simulink model "shuntconverterlms1"  (R2018a)
settings: Solver=VariableStepAuto  StartTime=0.0  StopTime=1  RelTol=1e-3
libraries: powerlib x20, eeGeneralControl x4, simulink x2
settings Model: Creator=sanje  LastModifiedBy=sanje
settings DataIOCC: ReturnWorkspaceOutputs=on
settings SFSimCC: SimUseLocalCustomCode=on
settings RTWCC: RTWUseLocalCustomCode=on

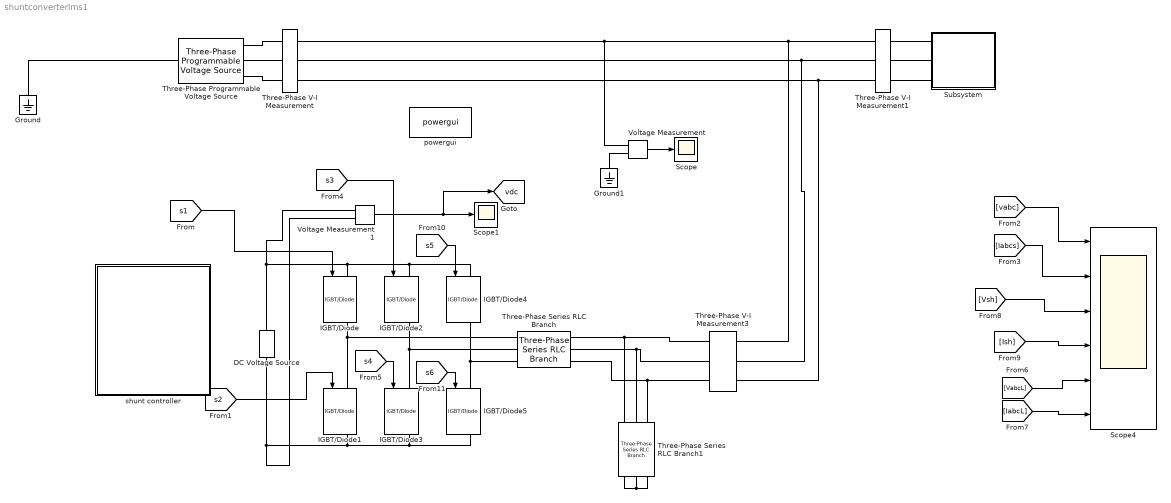
== system shuntconverterlms1 ==
  DC Voltage Source : powerlib/Electrical Sources/DC Voltage Source  Amplitude=700  Measurements=None
      settings: SourceProductName=Simscape Electrical
  Ground : powerlib/Elements/Ground  LConnTagsString=a
      settings: SourceProductName=Simscape Electrical
  Ground1 : powerlib/Elements/Ground  LConnTagsString=a
      settings: SourceProductName=Simscape Electrical
  IGBT/Diode{,1..5} (6 alike) : powerlib/Power Electronics/IGBT//Diode  Ron=1e-3  Rs=1e5  Cs=inf  Measurements=on
      settings: SourceProductName=Simscape Electrical
  Scope : Scope
  Scope1 : Scope
  Scope4 : Scope  NumInputPorts=6
  Subsystem : Subsystem
  Three-Phase Programmable Voltage Source : powerlib/Electrical Sources/Three-Phase Programmable Voltage Source  PositiveSequence="[415  0 50]"  VariationEntity=None  VariationType=Table of time-amplitude pairs  VariationTypeAlt=Step  VariationStep=0.5  VariationRate=10  VariationMagnitude=0.3  VariationFrequency=2  VariationTiming=[1 2]  VariationPhaseA=off  Amplitudes=[1 0.8 1 1.2 1.0]  TimeValues=[0 0.1 0.15 0.2 0.25]  HarmonicGeneration=off  HarmonicA=[3 0.2 -25 0]  HarmonicB=[2 0.15 35 2]  Timing="[0.05  3]"  BusType=swing  Pref=0  Qref=0  Qmin=-inf  Qmax=inf
      settings: SourceProductName=Simscape Electrical
  Three-Phase Series RLC Branch : powerlib/Elements/Three-Phase Series RLC Branch  LConnTagsString=A|B|C  RConnTagsString=A|B|C  BranchType=L  Resistance=1  Inductance=2.5e-3  Capacitance=1e-6  Measurements=None
      settings: SourceProductName=Simscape Electrical
  Three-Phase Series RLC Branch1 : powerlib/Elements/Three-Phase Series RLC Branch  LConnTagsString=A|B|C  RConnTagsString=A|B|C  BranchType=RC  Resistance=5  Inductance=1e-3  Capacitance=10e-6  Measurements=None
      settings: SourceProductName=Simscape Electrical
  Three-Phase V-I Measurement : powerlib/Measurements/Three-Phase V-I Measurement  VoltageMeasurement=phase-to-ground  SetLabelV=on  LabelV=vabc  Vpu=off  VpuLL=off  CurrentMeasurement=yes  SetLabelI=on  LabelI=Iabcs  Ipu=off  Pbase=100e6  Vbase=500e3  OutputType=Complex  PhasorSimulation=off  PSBequivalent=0
      settings: SourceProductName=Simscape Electrical
  Three-Phase V-I Measurement1 : powerlib/Measurements/Three-Phase V-I Measurement  VoltageMeasurement=phase-to-ground  SetLabelV=on  LabelV=VabcL  Vpu=off  VpuLL=off  CurrentMeasurement=yes  SetLabelI=on  LabelI=IabcL  Ipu=off  Pbase=100e6  Vbase=500e3  OutputType=Complex  PhasorSimulation=off  PSBequivalent=0
      settings: SourceProductName=Simscape Electrical
  Three-Phase V-I Measurement3 : powerlib/Measurements/Three-Phase V-I Measurement  VoltageMeasurement=phase-to-ground  SetLabelV=on  LabelV=Vsh  Vpu=off  VpuLL=off  CurrentMeasurement=yes  SetLabelI=on  LabelI=Ish  Ipu=off  Pbase=100e6  Vbase=500e3  OutputType=Complex  PhasorSimulation=off  PSBequivalent=0
      settings: SourceProductName=Simscape Electrical
  Voltage Measurement : powerlib/Measurements/Voltage Measurement  PhasorSimulation=off  OutputType=Complex  PSBequivalent=0
      settings: SourceProductName=Simscape Electrical
  Voltage Measurement1 : powerlib/Measurements/Voltage Measurement  PhasorSimulation=off  OutputType=Complex  PSBequivalent=0
      settings: SourceProductName=Simscape Electrical
  powergui : powerlib/powergui  Priority=1  SimulationMode=Discrete  SampleTime=10e-6  frequency=60  Iterations=50  frequencyindice=0  Pbase=100e6  ErrMax=1e-4  UnitsV=kV  UnitsW=MW  buscounter=0  FunctionMessages=off  echomessages=off  EnableUseOfTLC=off  CurrentSourceSwitches=off  DisableSnubberDevices=off  DisableRonSwitches=off  DisableVfSwitches=off  DisplayEquations=off  AutomaticDiscreteSolvers=off  SolverType=Tustin/Backward Euler (TBE)  Interpol=off  ExternalGateDelay=off  methode=off  Ts=100  x0status=blocks  SPID=on  SwTol=0  HookPort=off  NonlinearTolerance=1e-4  nMaxIteration=100  ContinueOnMaxIteration=off  RestoreLinks=warning  ResistiveCurrentMeasurement=off  Frange=[0:2:500]  Ylog=off  Xlog=on  ShowGrid=off  save=off  variable=ZData  structure=0  ZoomFFT=off  StartTime=0.0  cycles=1  DisplayStyle=1  fundamental=60  FreqAxis=off  MaxFrequency=1000  frequencyindicesteady=1  RmsSteady=1  display=off
      settings: SourceProductName=Simscape Electrical
  shunt controller : Subsystem
  tag scope: vdc=global
  wires:
  [Iabcs] -> Scope4/2
  [vabc] -> Scope4/1
  Voltage Measurement/1 -> Scope/1
  Voltage Measurement1/1 -> Scope1/1, [vdc]
  [Vsh] -> Scope4/3
  [VabcL] -> Scope4/5
  [IabcL] -> Scope4/6
  [Ish] -> Scope4/4
  [s1] -> IGBT/Diode/1
  [s2] -> IGBT/Diode1/1
  [s3] -> IGBT/Diode2/1
  [s4] -> IGBT/Diode3/1
  [s5] -> IGBT/Diode4/1
  [s6] -> IGBT/Diode5/1
  connections:
  Three-Phase Programmable Voltage Source/RConn1 -- Three-Phase V-I Measurement/LConn1
  Subsystem/LConn1 -- Three-Phase V-I Measurement1/RConn1
  Subsystem/LConn3 -- Three-Phase V-I Measurement1/RConn3
  Subsystem/LConn2 -- Three-Phase V-I Measurement1/RConn2
  Three-Phase Programmable Voltage Source/RConn3 -- Three-Phase V-I Measurement/LConn3
  Ground/LConn1 -- Three-Phase Programmable Voltage Source/LConn1
  Three-Phase V-I Measurement/LConn2 -- Three-Phase Programmable Voltage Source/RConn2
  Three-Phase V-I Measurement1/LConn1 -- Three-Phase V-I Measurement3/RConn1 -- Voltage Measurement/LConn1 -- Three-Phase V-I Measurement/RConn1
  Three-Phase V-I Measurement1/LConn2 -- Three-Phase V-I Measurement3/RConn2 -- Three-Phase V-I Measurement/RConn2
  Three-Phase V-I Measurement1/LConn3 -- Three-Phase V-I Measurement3/RConn3 -- Three-Phase V-I Measurement/RConn3
  Three-Phase Series RLC Branch/LConn2 -- Three-Phase Series RLC Branch1/RConn2 -- Three-Phase V-I Measurement3/LConn2
  Three-Phase Series RLC Branch/LConn3 -- Three-Phase Series RLC Branch1/RConn3 -- Three-Phase V-I Measurement3/LConn3
  Three-Phase Series RLC Branch/LConn1 -- Three-Phase Series RLC Branch1/RConn1 -- Three-Phase V-I Measurement3/LConn1
  Ground1/LConn1 -- Voltage Measurement/LConn2
  Three-Phase Series RLC Branch1/LConn1 -- Three-Phase Series RLC Branch1/LConn3 -- Three-Phase Series RLC Branch1/LConn2
  IGBT/Diode1/LConn1 -- Three-Phase Series RLC Branch/RConn1 -- IGBT/Diode/RConn1
  IGBT/Diode4/RConn1 -- IGBT/Diode5/LConn1 -- Three-Phase Series RLC Branch/RConn3
  IGBT/Diode2/RConn1 -- IGBT/Diode3/LConn1 -- Three-Phase Series RLC Branch/RConn2
  DC Voltage Source/RConn1 -- IGBT/Diode4/LConn1 -- IGBT/Diode2/LConn1 -- IGBT/Diode/LConn1 -- Voltage Measurement1/LConn1
  DC Voltage Source/LConn1 -- Voltage Measurement1/LConn2 -- IGBT/Diode5/RConn1 -- IGBT/Diode3/RConn1 -- IGBT/Diode1/RConn1

== system shuntconverterlms1/Subsystem ==
  Series RLC Branch11 : powerlib/Elements/Series RLC Branch  LConnTagsString=__new0  RConnTagsString=__new0  BranchType=RL  Resistance=11  Inductance=120e-3  SetiL0=off  InitialCurrent=0  Capacitance=1e-6  Setx0=off  InitialVoltage=0  Measurements=None
      settings: SourceProductName=Simscape Electrical
  Universal Bridge : powerlib/Power Electronics/Universal Bridge  Arms=3  SnubberResistance=1e5  SnubberCapacitance=inf  Device=Diodes  Ron=1e-3  Lon=0  ForwardVoltages="[  0  0  ]"  ForwardVoltage=0  GTOparameters=[ 10e-6 , 20e-6 ]  IGBTparameters=[ 1e-6 , 2e-6 ]  Measurements=None  Measurements_2=None  converterType=Rectifier
      settings: SourceProductName=Simscape Electrical
  Conn1 : PMIOPort  Side=Left
  Conn4 : PMIOPort  Port=2  Side=Left
  Conn2 : PMIOPort  Port=3  Side=Left
  connections:
  Universal Bridge/RConn2 -- Series RLC Branch11/RConn1
  Universal Bridge/RConn1 -- Series RLC Branch11/LConn1
  Conn1/RConn1 -- Universal Bridge/LConn1
  Conn2/RConn1 -- Universal Bridge/LConn3
  Universal Bridge/LConn2 -- Conn4/RConn1

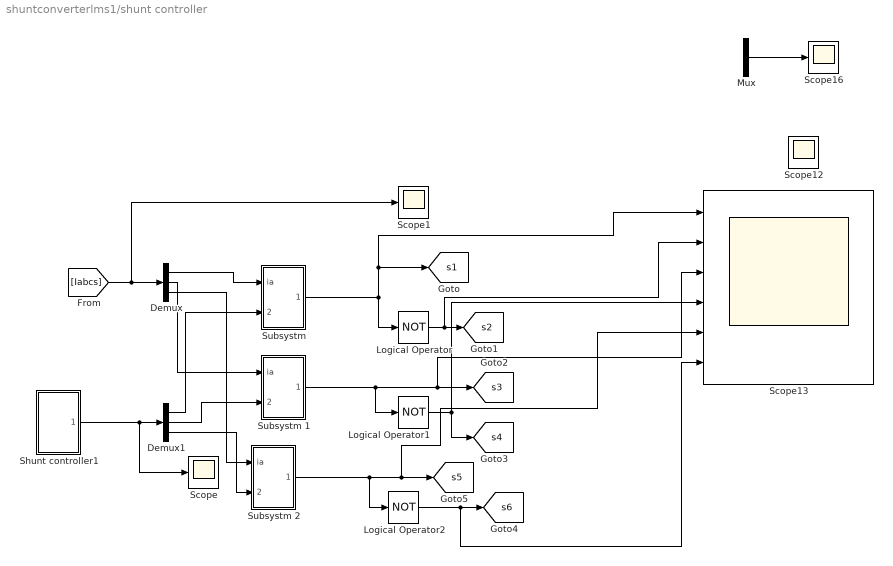
== system shuntconverterlms1/shunt controller ==
  Demux : Demux  Outputs=3
  Demux1 : Demux  Outputs=3
  Logical Operator : Logic  Operator=NOT  AllPortsSameDT=off  OutDataTypeStr=boolean
  Logical Operator1 : Logic  Operator=NOT  AllPortsSameDT=off  OutDataTypeStr=boolean
  Logical Operator2 : Logic  Operator=NOT  AllPortsSameDT=off  OutDataTypeStr=boolean
  Mux : Mux  Inputs=3
  Scope{,1,12,16} (4 alike) : Scope
  Scope13 : Scope  NumInputPorts=6
  Shunt controller1 : Subsystem
  "Subsystm " : Subsystem
  Subsystm 1 : Subsystem
  Subsystm 2 : Subsystem
  tag scope: s1=global, s2=global, s3=global, s4=global, s5=global, s6=global
  wires:
  Mux/1 -> Scope16/1
  Shunt controller1/1(Outport) -> Scope/1, Demux1/1
  [Iabcs] -> Scope1/1, Demux/1
  Demux/1 -> "Subsystm "/1(ia)
  Demux1/1 -> "Subsystm "/2(In2)
  Demux/2 -> Subsystm 1/1(ia)
  Demux1/2 -> Subsystm 1/2(In2)
  Demux/3 -> Subsystm 2/1(ia)
  Demux1/3 -> Subsystm 2/2(In2)
  "Subsystm "/1(Out1) -> Logical Operator/1, Scope13/1, [s1]
  Subsystm 1/1(Out1) -> Scope13/3, [s3], Logical Operator1/1
  Subsystm 2/1(Out1) -> Scope13/5, [s5], Logical Operator2/1
  Logical Operator/1 -> Scope13/2, [s2]
  Logical Operator1/1 -> [s4], Scope13/4
  Logical Operator2/1 -> Scope13/6, [s6]

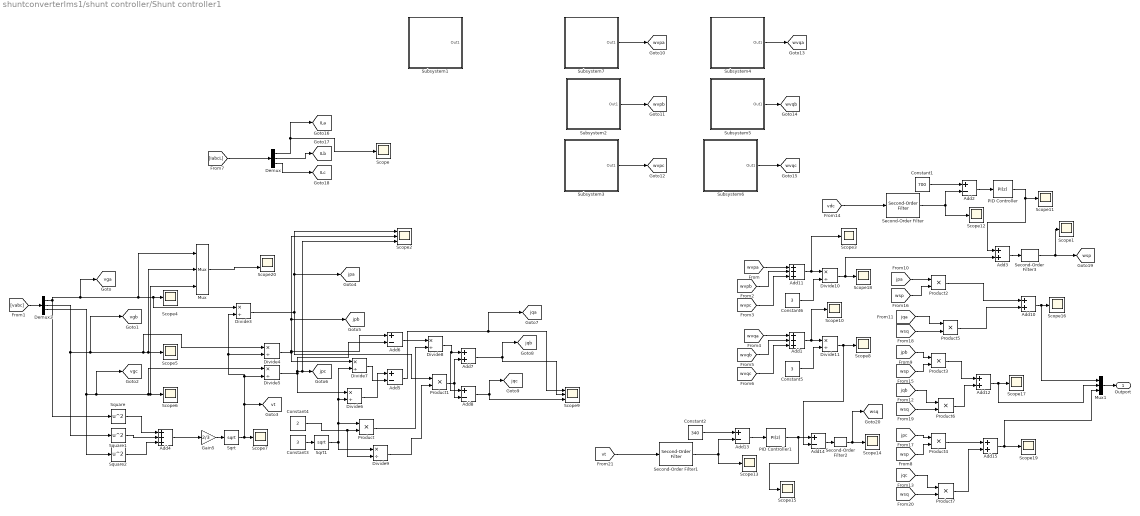
== system shuntconverterlms1/shunt controller/Shunt controller1 ==
  Add1 : Sum  Inputs=+++
  Add{3,7,10,12,15} (5 alike) : Sum
  Add11 : Sum  Inputs=+++
  Add{2,5..6,8,13..14} (6 alike) : Sum  Inputs=+-
  Add4 : Sum  Inputs=+++
  Constant1 : Constant  Value=700
  Constant2 : Constant  Value=340
  Constant3 : Constant  Value=3
  Constant4 : Constant  Value=2
  Constant5 : Constant  Value=3
  Constant6 : Constant  Value=3
  Demux : Demux  Outputs=3
  Demux2 : Demux  Outputs=3
  Divide{3..11} (9 alike) : Product  Inputs=*/
  Gain5 : Gain  Gain=2/3
  Mux : Mux  Inputs=3
  Mux1 : Mux  Inputs=3
  PID Controller : simulink/Continuous/PID Controller  Controller=PI  Form=Parallel  TimeDomain=Discrete-time  SampleTime=-1  IntegratorMethod=Forward Euler  FilterMethod=Forward Euler  ControllerParametersSource=internal  P=1  I=1  D=0  UseFilter=on  N=100  TunerSelectOption=Transfer Function Based (PID Tuner App)  InitialConditionSource=internal  InitialConditionForIntegrator=0  InitialConditionForFilter=0  DifferentiatorICPrevScaledInput=0  ExternalReset=none  TrackingMode=off  Kt=1  LimitOutput=off  UpperSaturationLimit=inf  LowerSaturationLimit=-inf  LinearizeAsGain=on  AntiWindupMode=none  Kb=1  POutMin=[]  POutMax=[]  IOutMin=[]  IOutMax=[]  DOutMin=[]  DOutMax=[]  NOutMin=[]  NOutMax=[]  SumOutMin=[]  SumOutMax=[]  SaturationOutMin=[]  SaturationOutMax=[]  PParamMin=[]  PParamMax=[]  IParamMin=[]  IParamMax=[]  DParamMin=[]  DParamMax=[]  NParamMin=[]  NParamMax=[]  KbParamMin=[]  KbParamMax=[]  KtParamMin=[]  KtParamMax=[]  KbOutMin=[]  KbOutMax=[]  KtOutMin=[]  KtOutMax=[]  IntegratorOutMin=[]  IntegratorOutMax=[]  FilterOutMin=[]  FilterOutMax=[]  SumI1OutMin=[]  SumI1OutMax=[]  SumI2OutMin=[]  SumI2OutMax=[]  SumI3OutMin=[]  SumI3OutMax=[]  SumDOutMin=[]  SumDOutMax=[]  DifferentiatorOutMin=[]  DifferentiatorOutMax=[]  FilterDiffOutCoefMin=[]  FilterDiffOutCoefMax=[]  ReciprocalOutMin=[]  ReciprocalOutMax=[]  SumDenOutMin=[]  SumDenOutMax=[]  SumNumOutMin=[]  SumNumOutMax=[]  DivideOutMin=[]  DivideOutMax=[]  IntegratorContinuousStateAttributes=''  IntegratorStateMustResolveToSignalObject=off  IntegratorRTWStateStorageClass=Auto  FilterContinuousStateAttributes=''  FilterStateMustResolveToSignalObject=off  FilterRTWStateStorageClass=Auto
  PID Controller1 : simulink/Continuous/PID Controller  Controller=PI  Form=Parallel  TimeDomain=Discrete-time  SampleTime=-1  IntegratorMethod=Forward Euler  FilterMethod=Forward Euler  ControllerParametersSource=internal  P=1  I=1  D=0  UseFilter=on  N=100  TunerSelectOption=Transfer Function Based (PID Tuner App)  InitialConditionSource=internal  InitialConditionForIntegrator=0  InitialConditionForFilter=0  DifferentiatorICPrevScaledInput=0  ExternalReset=none  TrackingMode=off  Kt=1  LimitOutput=off  UpperSaturationLimit=inf  LowerSaturationLimit=-inf  LinearizeAsGain=on  AntiWindupMode=none  Kb=1  POutMin=[]  POutMax=[]  IOutMin=[]  IOutMax=[]  DOutMin=[]  DOutMax=[]  NOutMin=[]  NOutMax=[]  SumOutMin=[]  SumOutMax=[]  SaturationOutMin=[]  SaturationOutMax=[]  PParamMin=[]  PParamMax=[]  IParamMin=[]  IParamMax=[]  DParamMin=[]  DParamMax=[]  NParamMin=[]  NParamMax=[]  KbParamMin=[]  KbParamMax=[]  KtParamMin=[]  KtParamMax=[]  KbOutMin=[]  KbOutMax=[]  KtOutMin=[]  KtOutMax=[]  IntegratorOutMin=[]  IntegratorOutMax=[]  FilterOutMin=[]  FilterOutMax=[]  SumI1OutMin=[]  SumI1OutMax=[]  SumI2OutMin=[]  SumI2OutMax=[]  SumI3OutMin=[]  SumI3OutMax=[]  SumDOutMin=[]  SumDOutMax=[]  DifferentiatorOutMin=[]  DifferentiatorOutMax=[]  FilterDiffOutCoefMin=[]  FilterDiffOutCoefMax=[]  ReciprocalOutMin=[]  ReciprocalOutMax=[]  SumDenOutMin=[]  SumDenOutMax=[]  SumNumOutMin=[]  SumNumOutMax=[]  DivideOutMin=[]  DivideOutMax=[]  IntegratorContinuousStateAttributes=''  IntegratorStateMustResolveToSignalObject=off  IntegratorRTWStateStorageClass=Auto  FilterContinuousStateAttributes=''  FilterStateMustResolveToSignalObject=off  FilterRTWStateStorageClass=Auto
  Product{,1..7} (8 alike) : Product
  Scope{,1,3..8,10..19} (18 alike) : Scope
  Scope2 : Scope  NumInputPorts=3
  Scope20 : Scope  NumInputPorts=2
  Scope9 : Scope  NumInputPorts=3
  Second-Order Filter : eeGeneralControl/Second-Order Filter  FilterType=Low-pass  fn=50  Zeta=0.707  Ts=10e-6  A0=0  Ph0=0  f0=0  b0=0
      settings: SourceProductName=Simscape Electrical  SourceProductBaseCode=PS
  Second-Order Filter1 : eeGeneralControl/Second-Order Filter  FilterType=Low-pass  fn=50  Zeta=0.707  Ts=10e-6  A0=0  Ph0=0  f0=0  b0=0
      settings: SourceProductName=Simscape Electrical  SourceProductBaseCode=PS
  Second-Order Filter2 : eeGeneralControl/Second-Order Filter  FilterType=Low-pass  fn=10  Zeta=0.707  Ts=10e-6  A0=0  Ph0=0  f0=0  b0=0
      settings: SourceProductName=Simscape Electrical  SourceProductBaseCode=PS
  Second-Order Filter3 : eeGeneralControl/Second-Order Filter  FilterType=Low-pass  fn=10  Zeta=0.707  Ts=10e-6  A0=0  Ph0=0  f0=0  b0=0
      settings: SourceProductName=Simscape Electrical  SourceProductBaseCode=PS
  Sqrt : Sqrt  SaturateOnIntegerOverflow=on
  Sqrt1 : Sqrt  SaturateOnIntegerOverflow=on
  Square : Math  Operator=square  SaturateOnIntegerOverflow=on
  Square1 : Math  Operator=square  SaturateOnIntegerOverflow=on
  Square2 : Math  Operator=square  SaturateOnIntegerOverflow=on
  Subsystem1 : Subsystem
  Subsystem2 : Subsystem
  Subsystem3 : Subsystem
  Subsystem4 : Subsystem
  Subsystem5 : Subsystem
  Subsystem6 : Subsystem
  Subsystem7 : Subsystem
  Outport : Outport
  tag scope: ILa=global, ILb=global, ILc=global, jpa=global, jpb=global, jpc=global, jqa=global, jqb=global, jqc=global, vga=global, vgb=global, vgc=global, vt=global, wsp=global, wsq=global, wvpa=global, wvpb=global, wvpc=global, wvqa=global, wvqb=global, wvqc=global
  wires:
  Add6/1 -> Divide8/1
  Constant4/1 -> Divide9/2, Product/2
  Constant3/1 -> Sqrt1/1
  Add8/1 -> [jqc], Scope9/3
  Product/1 -> Divide8/2
  Divide5/1 -> Add6/2, Scope2/3, [jpc], Divide6/1
  Divide4/1 -> Divide7/1, Scope2/2, [jpb], Add6/1
  Square1/1 -> Add4/2
  Add7/1 -> [jqb], Scope9/2
  Divide8/1 -> Add7/1, Add8/1
  Product1/1 -> Add8/2, Add7/2
  Mux/1 -> Scope20/2
  Divide7/1 -> Add5/2
  Divide9/1 -> Product1/2
  Sqrt1/1 -> Product/1, Divide7/2, Divide6/2, Divide9/1
  Divide6/1 -> Add5/1
  Square/1 -> Add4/1
  Add4/1 -> Gain5/1
  Sqrt/1 -> Divide5/2, Divide4/2, Divide3/2, [vt], Scope7/1
  Gain5/1 -> Sqrt/1
  Divide3/1 -> Product1/1, Scope2/1, [jpa]
  Demux2/2 -> Square1/1, [vgb], Mux/2, Scope5/1, Divide4/1
  Demux2/1 -> [vga], Mux/1, Divide3/1, Scope4/1, Square/1
  Square2/1 -> Add4/3
  Demux2/3 -> Square2/1, [vgc], Mux/3, Scope6/1, Divide5/1
  Add5/1 -> [jqa], Scope9/1
  [vabc] -> Demux2/1
  [wvpb] -> Add11/2
  [wvqa] -> Add1/1
  [wvqb] -> Add1/2
  Subsystem4/1(Out1) -> [wvqa]
  Subsystem3/1(Out1) -> [wvpc]
  [wvqc] -> Add1/3
  [wvpc] -> Add11/3
  Add11/1 -> Scope3/1, Divide10/1
  Add1/1 -> Scope10/1, Divide11/1
  Subsystem5/1(Out1) -> [wvqb]
  Divide10/1 -> Add3/2, Scope18/1
  Subsystem2/1(Out1) -> [wvpb]
  [wvpa] -> Add11/1
  Constant6/1 -> Divide10/2
  Subsystem7/1(Out1) -> [wvpa]
  Constant5/1 -> Divide11/2
  Subsystem6/1(Out1) -> [wvqc]
  Divide11/1 -> Add14/2, Scope8/1
  [IabcL] -> Demux/1
  Demux/1 -> [ILa], Scope/1
  Demux/2 -> [ILb]
  Demux/3 -> [ILc]
  Constant1/1 -> Add2/1
  [vdc] -> Second-Order Filter/1
  Second-Order Filter/1 -> Add2/2, Scope12/1
  Add2/1 -> PID Controller/1
  PID Controller/1 -> Add3/1, Scope11/1
  [jpa] -> Product2/1
  [wsp] -> Product2/2
  [jpb] -> Product3/1
  [wsp] -> Product3/2
  [jpc] -> Product4/1
  [wsp] -> Product4/2
  [wsq] -> Product5/2
  [jqa] -> Product5/1
  [jqb] -> Product6/1
  [wsq] -> Product6/2
  [wsq] -> Product7/2
  [jqc] -> Product7/1
  Product2/1 -> Add10/1
  Product5/1 -> Add10/2
  Product3/1 -> Add12/1
  Product6/1 -> Add12/2
  PID Controller1/1 -> Scope15/1, Add14/1
  Add13/1 -> PID Controller1/1
  Second-Order Filter1/1 -> Scope13/1, Add13/2
  [vt] -> Second-Order Filter1/1
  Constant2/1 -> Add13/1
  Add14/1 -> Second-Order Filter2/1
  Product4/1 -> Add15/1
  Product7/1 -> Add15/2
  Add10/1 -> Mux1/1, Scope16/1
  Add12/1 -> Mux1/2, Scope17/1
  Add15/1 -> Mux1/3, Scope19/1
  Mux1/1 -> Outport/1
  Second-Order Filter2/1 -> [wsq], Scope14/1
  Add3/1 -> Second-Order Filter3/1
  Second-Order Filter3/1 -> Scope1/1, [wsp]

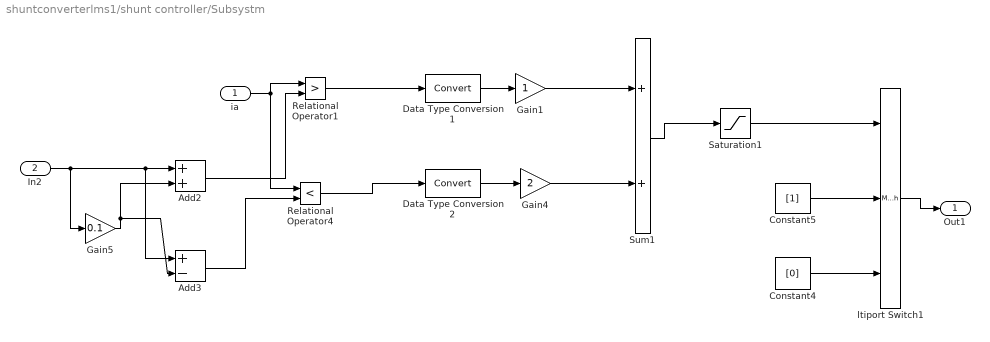
== system shuntconverterlms1/shunt controller/Subsystm  ==
  ia : Inport
  In2 : Inport  Port=2
  Add2 : Sum
  Add3 : Sum  Inputs=+-
  Constant4 : Constant  Value=[0]
  Constant5 : Constant  Value=[1]
  Data Type Conversion1 : DataTypeConversion  SaturateOnIntegerOverflow=on  RndMeth=Zero
  Data Type Conversion2 : DataTypeConversion  SaturateOnIntegerOverflow=on  RndMeth=Zero
  Gain1 : Gain  SaturateOnIntegerOverflow=on  OutDataTypeStr=Inherit: Same as input  ParamDataTypeStr=Inherit: Same as input
  Gain4 : Gain  Gain=2  SaturateOnIntegerOverflow=on  OutDataTypeStr=Inherit: Same as input  ParamDataTypeStr=Inherit: Same as input
  Gain5 : Gain  Gain=0.1
  Relational Operator1 : RelationalOperator  Operator=>  RndMeth=Nearest  InputSameDT=on
  Relational Operator4 : RelationalOperator  Operator=<  RndMeth=Nearest  InputSameDT=on
  Saturation1 : Saturate  UpperLimit=2  LowerLimit=1
  Sum1 : Sum  SaturateOnIntegerOverflow=on  InputSameDT=on  OutDataTypeStr=Inherit: Same as first input
  ltiport Switch1 : MultiPortSwitch  Inputs=2
  Out1 : Outport
  wires:
  In2/1 -> Add3/1, Add2/1, Gain5/1
  Data Type Conversion2/1 -> Gain4/1
  Data Type Conversion1/1 -> Gain1/1
  Relational Operator1/1 -> Data Type Conversion1/1
  Relational Operator4/1 -> Data Type Conversion2/1
  ia/1 -> Relational Operator4/1, Relational Operator1/1
  Gain5/1 -> Add2/2, Add3/2
  Add2/1 -> Relational Operator1/2
  Add3/1 -> Relational Operator4/2
  Saturation1/1 -> ltiport Switch1/1
  Constant5/1 -> ltiport Switch1/2
  Constant4/1 -> ltiport Switch1/3
  Gain1/1 -> Sum1/1
  Gain4/1 -> Sum1/2
  Sum1/1 -> Saturation1/1
  ltiport Switch1/1 -> Out1/1

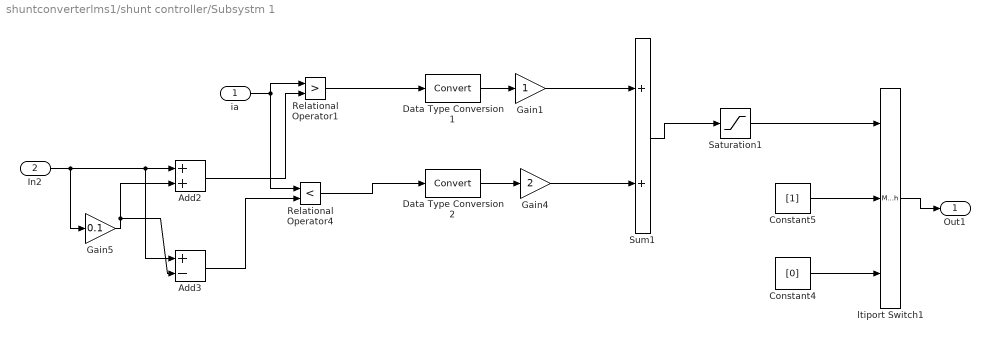
== system shuntconverterlms1/shunt controller/Subsystm 1 ==
  ia : Inport
  In2 : Inport  Port=2
  Add2 : Sum
  Add3 : Sum  Inputs=+-
  Constant4 : Constant  Value=[0]
  Constant5 : Constant  Value=[1]
  Data Type Conversion1 : DataTypeConversion  SaturateOnIntegerOverflow=on  RndMeth=Zero
  Data Type Conversion2 : DataTypeConversion  SaturateOnIntegerOverflow=on  RndMeth=Zero
  Gain1 : Gain  SaturateOnIntegerOverflow=on  OutDataTypeStr=Inherit: Same as input  ParamDataTypeStr=Inherit: Same as input
  Gain4 : Gain  Gain=2  SaturateOnIntegerOverflow=on  OutDataTypeStr=Inherit: Same as input  ParamDataTypeStr=Inherit: Same as input
  Gain5 : Gain  Gain=0.1
  Relational Operator1 : RelationalOperator  Operator=>  RndMeth=Nearest  InputSameDT=on
  Relational Operator4 : RelationalOperator  Operator=<  RndMeth=Nearest  InputSameDT=on
  Saturation1 : Saturate  UpperLimit=2  LowerLimit=1
  Sum1 : Sum  SaturateOnIntegerOverflow=on  InputSameDT=on  OutDataTypeStr=Inherit: Same as first input
  ltiport Switch1 : MultiPortSwitch  Inputs=2
  Out1 : Outport
  wires:
  ltiport Switch1/1 -> Out1/1
  Sum1/1 -> Saturation1/1
  Gain4/1 -> Sum1/2
  Gain1/1 -> Sum1/1
  Constant4/1 -> ltiport Switch1/3
  Constant5/1 -> ltiport Switch1/2
  Saturation1/1 -> ltiport Switch1/1
  Add3/1 -> Relational Operator4/2
  Add2/1 -> Relational Operator1/2
  Gain5/1 -> Add3/2, Add2/2
  ia/1 -> Relational Operator1/1, Relational Operator4/1
  Relational Operator4/1 -> Data Type Conversion2/1
  Relational Operator1/1 -> Data Type Conversion1/1
  Data Type Conversion1/1 -> Gain1/1
  Data Type Conversion2/1 -> Gain4/1
  In2/1 -> Gain5/1, Add2/1, Add3/1

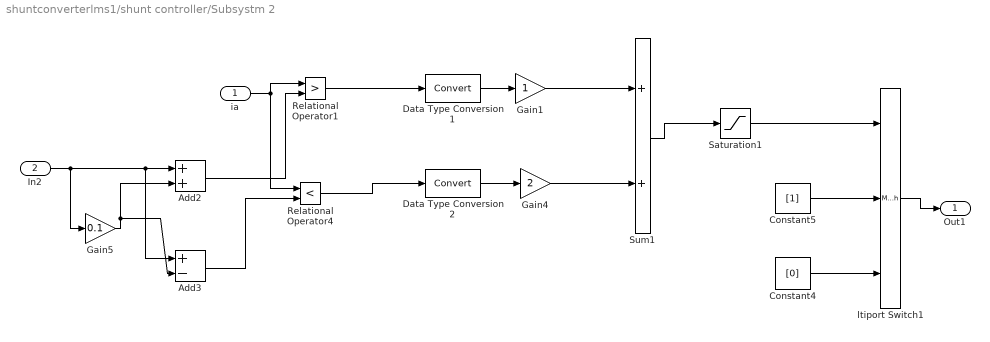
== system shuntconverterlms1/shunt controller/Subsystm 2 ==
  ia : Inport
  In2 : Inport  Port=2
  Add2 : Sum
  Add3 : Sum  Inputs=+-
  Constant4 : Constant  Value=[0]
  Constant5 : Constant  Value=[1]
  Data Type Conversion1 : DataTypeConversion  SaturateOnIntegerOverflow=on  RndMeth=Zero
  Data Type Conversion2 : DataTypeConversion  SaturateOnIntegerOverflow=on  RndMeth=Zero
  Gain1 : Gain  SaturateOnIntegerOverflow=on  OutDataTypeStr=Inherit: Same as input  ParamDataTypeStr=Inherit: Same as input
  Gain4 : Gain  Gain=2  SaturateOnIntegerOverflow=on  OutDataTypeStr=Inherit: Same as input  ParamDataTypeStr=Inherit: Same as input
  Gain5 : Gain  Gain=0.1
  Relational Operator1 : RelationalOperator  Operator=>  RndMeth=Nearest  InputSameDT=on
  Relational Operator4 : RelationalOperator  Operator=<  RndMeth=Nearest  InputSameDT=on
  Saturation1 : Saturate  UpperLimit=2  LowerLimit=1
  Sum1 : Sum  SaturateOnIntegerOverflow=on  InputSameDT=on  OutDataTypeStr=Inherit: Same as first input
  ltiport Switch1 : MultiPortSwitch  Inputs=2
  Out1 : Outport
  wires:
  In2/1 -> Add3/1, Add2/1, Gain5/1
  Data Type Conversion2/1 -> Gain4/1
  Data Type Conversion1/1 -> Gain1/1
  Relational Operator1/1 -> Data Type Conversion1/1
  Relational Operator4/1 -> Data Type Conversion2/1
  ia/1 -> Relational Operator4/1, Relational Operator1/1
  Gain5/1 -> Add2/2, Add3/2
  Add2/1 -> Relational Operator1/2
  Add3/1 -> Relational Operator4/2
  Saturation1/1 -> ltiport Switch1/1
  Constant5/1 -> ltiport Switch1/2
  Constant4/1 -> ltiport Switch1/3
  Gain1/1 -> Sum1/1
  Gain4/1 -> Sum1/2
  Sum1/1 -> Saturation1/1
  ltiport Switch1/1 -> Out1/1

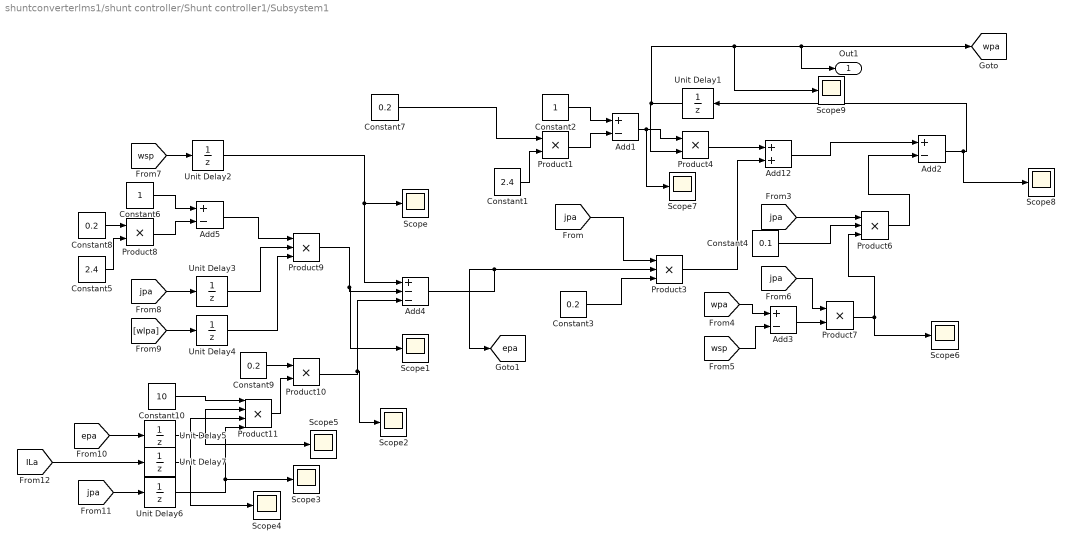
== system shuntconverterlms1/shunt controller/Shunt controller1/Subsystem1 ==
  Add{1..3,5} (4 alike) : Sum  Inputs=+-
  Add12 : Sum
  Add4 : Sum  Inputs=+--
  Constant1 : Constant  Value=2.4
  Constant10 : Constant  Value=10
  Constant2 : Constant
  Constant{3,7..9} (4 alike) : Constant  Value=0.2
  Constant4 : Constant  Value=0.1
  Constant5 : Constant  Value=2.4
  Constant6 : Constant
  Product{1,4,7..8,10} (5 alike) : Product
  Product11 : Product  Inputs=4
  Product3 : Product  Inputs=3
  Product6 : Product  Inputs=3
  Product9 : Product  Inputs=3
  Scope{,1..9} (10 alike) : Scope
  Unit Delay{1..7} (7 alike) : UnitDelay  SampleTime=10e-6  HasFrameUpgradeWarning=on
  Out1 : Outport
  tag scope: epa=global, wpa=global
  wires:
  Constant7/1 -> Product1/1
  Constant1/1 -> Product1/2
  Constant2/1 -> Add1/1
  Product1/1 -> Add1/2
  Add1/1 -> Scope7/1, Product4/1
  Product4/1 -> Add12/1
  Add12/1 -> Add2/1
  [jpa] -> Product3/1
  Constant3/1 -> Product3/3
  Product3/1 -> Add12/2
  [jpa] -> Product6/1
  Product6/1 -> Add2/2
  Constant4/1 -> Product6/2
  [wpa] -> Add3/1
  [wsp] -> Add3/2
  Add3/1 -> Product7/2
  [jpa] -> Product7/1
  Product7/1 -> Product6/3, Scope6/1
  [wsp] -> Unit Delay2/1
  Unit Delay2/1 -> Scope/1, Add4/1
  Product8/1 -> Add5/2
  Constant6/1 -> Add5/1
  Constant5/1 -> Product8/2
  Constant8/1 -> Product8/1
  [jpa] -> Unit Delay3/1
  [wlpa] -> Unit Delay4/1
  Add5/1 -> Product9/1
  Unit Delay3/1 -> Product9/2
  Unit Delay4/1 -> Product9/3
  Constant9/1 -> Product10/1
  Add4/1 -> Product3/2, [epa]
  [epa] -> Unit Delay5/1
  [jpa] -> Unit Delay6/1
  Constant10/1 -> Product11/1
  Unit Delay6/1 -> Scope3/1, Product11/4
  [ILa] -> Unit Delay7/1
  Unit Delay7/1 -> Product11/3, Scope4/1
  Product11/1 -> Product10/2
  Product9/1 -> Scope1/1, Add4/2
  Product10/1 -> Scope2/1, Add4/3
  Unit Delay5/1 -> Scope5/1, Product11/2
  Add2/1 -> Scope8/1, Unit Delay1/1
  Unit Delay1/1 -> Scope9/1, Out1/1, [wpa], Product4/2

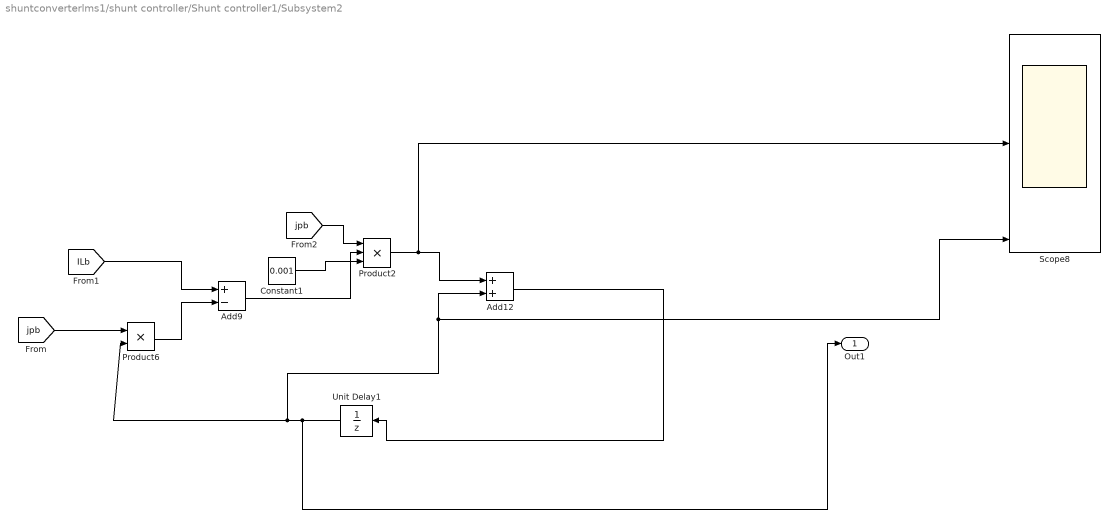
== system shuntconverterlms1/shunt controller/Shunt controller1/Subsystem2 ==
  Add12 : Sum
  Add9 : Sum  Inputs=+-
  Constant1 : Constant  Value=0.001
  Product2 : Product  Inputs=3
  Product6 : Product
  Scope8 : Scope  NumInputPorts=7
  Unit Delay1 : UnitDelay  SampleTime=10e-6  HasFrameUpgradeWarning=on
  Out1 : Outport
  wires:
  [jpb] -> Product2/1
  Product6/1 -> Add9/2
  Add9/1 -> Product2/2
  [jpb] -> Product6/1
  Add12/1 -> Unit Delay1/1
  Unit Delay1/1 -> Add12/2, Scope8/7, Product6/2, Out1/1
  Constant1/1 -> Product2/3
  [ILb] -> Add9/1
  Product2/1 -> Add12/1, Scope8/4

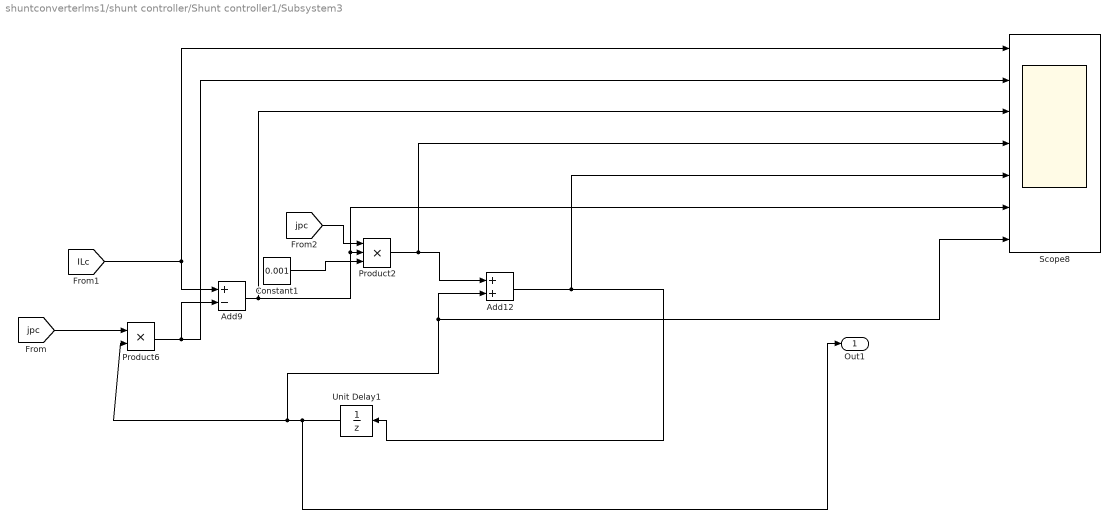
== system shuntconverterlms1/shunt controller/Shunt controller1/Subsystem3 ==
  Add12 : Sum
  Add9 : Sum  Inputs=+-
  Constant1 : Constant  Value=0.001
  Product2 : Product  Inputs=3
  Product6 : Product
  Scope8 : Scope  NumInputPorts=7
  Unit Delay1 : UnitDelay  SampleTime=10e-6  HasFrameUpgradeWarning=on
  Out1 : Outport
  wires:
  Product2/1 -> Scope8/4, Add12/1
  [ILc] -> Add9/1, Scope8/1
  Constant1/1 -> Product2/3
  Unit Delay1/1 -> Out1/1, Product6/2, Scope8/7, Add12/2
  Add12/1 -> Scope8/5, Unit Delay1/1
  [jpc] -> Product6/1
  Add9/1 -> Scope8/6, Product2/2, Scope8/3
  Product6/1 -> Scope8/2, Add9/2
  [jpc] -> Product2/1

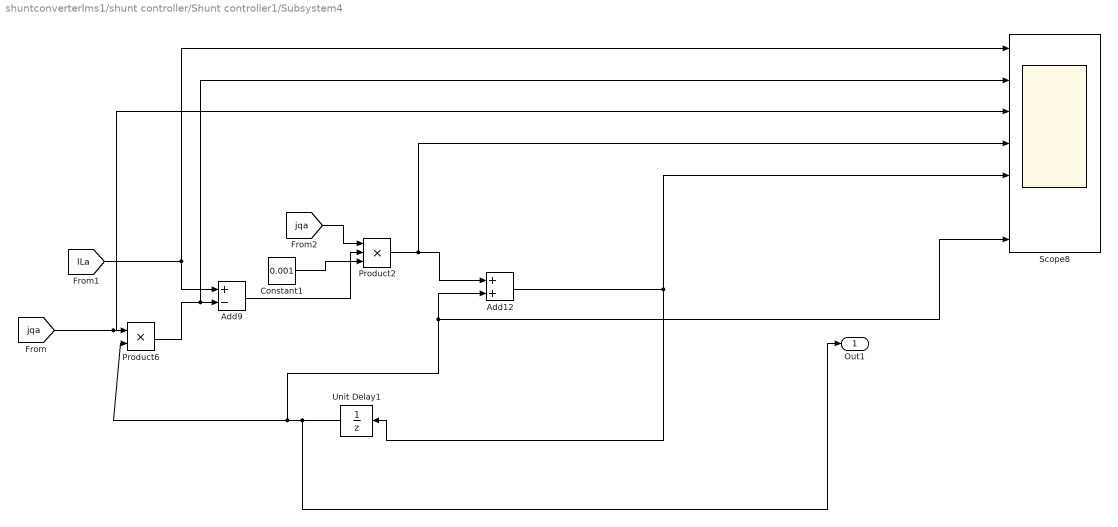
== system shuntconverterlms1/shunt controller/Shunt controller1/Subsystem4 ==
  Add12 : Sum
  Add9 : Sum  Inputs=+-
  Constant1 : Constant  Value=0.001
  Product2 : Product  Inputs=3
  Product6 : Product
  Scope8 : Scope  NumInputPorts=7
  Unit Delay1 : UnitDelay  SampleTime=10e-6  HasFrameUpgradeWarning=on
  Out1 : Outport
  wires:
  [jqa] -> Product2/1
  Product6/1 -> Scope8/2, Add9/2
  Add9/1 -> Product2/2
  [jqa] -> Scope8/3, Product6/1
  Add12/1 -> Unit Delay1/1, Scope8/5
  Unit Delay1/1 -> Add12/2, Scope8/7, Product6/2, Out1/1
  Constant1/1 -> Product2/3
  [ILa] -> Add9/1, Scope8/1
  Product2/1 -> Add12/1, Scope8/4

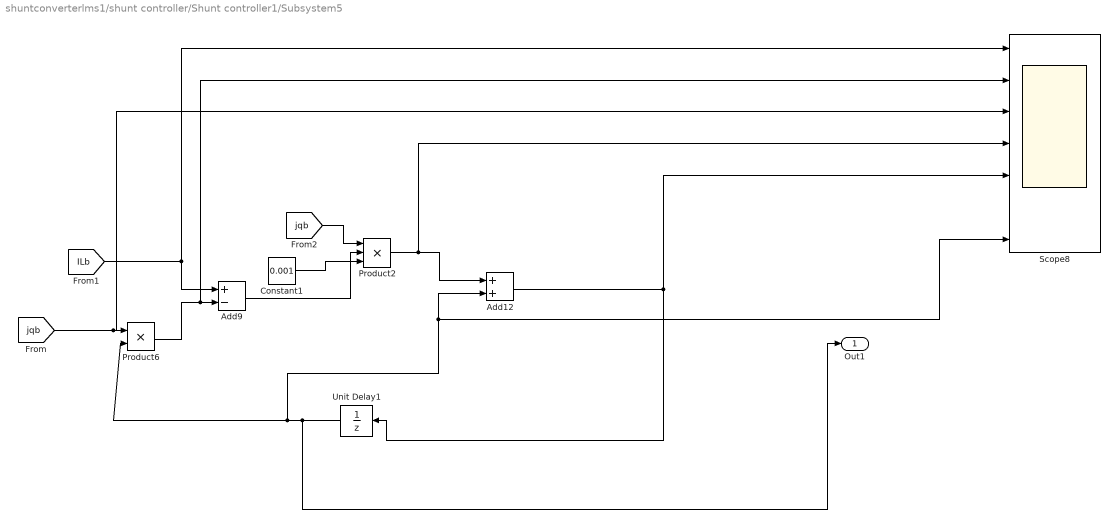
== system shuntconverterlms1/shunt controller/Shunt controller1/Subsystem5 ==
  Add12 : Sum
  Add9 : Sum  Inputs=+-
  Constant1 : Constant  Value=0.001
  Product2 : Product  Inputs=3
  Product6 : Product
  Scope8 : Scope  NumInputPorts=7
  Unit Delay1 : UnitDelay  SampleTime=10e-6  HasFrameUpgradeWarning=on
  Out1 : Outport
  wires:
  Product2/1 -> Scope8/4, Add12/1
  [ILb] -> Scope8/1, Add9/1
  Constant1/1 -> Product2/3
  Unit Delay1/1 -> Out1/1, Product6/2, Scope8/7, Add12/2
  Add12/1 -> Scope8/5, Unit Delay1/1
  [jqb] -> Product6/1, Scope8/3
  Add9/1 -> Product2/2
  Product6/1 -> Add9/2, Scope8/2
  [jqb] -> Product2/1

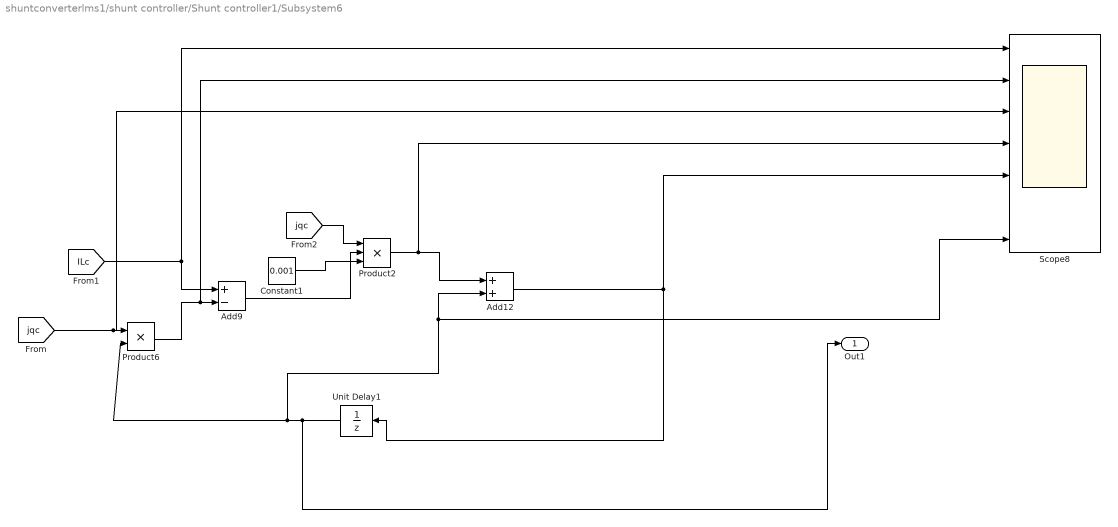
== system shuntconverterlms1/shunt controller/Shunt controller1/Subsystem6 ==
  Add12 : Sum
  Add9 : Sum  Inputs=+-
  Constant1 : Constant  Value=0.001
  Product2 : Product  Inputs=3
  Product6 : Product
  Scope8 : Scope  NumInputPorts=7
  Unit Delay1 : UnitDelay  SampleTime=10e-6  HasFrameUpgradeWarning=on
  Out1 : Outport
  wires:
  [jqc] -> Product2/1
  Product6/1 -> Scope8/2, Add9/2
  Add9/1 -> Product2/2
  [jqc] -> Scope8/3, Product6/1
  Add12/1 -> Unit Delay1/1, Scope8/5
  Unit Delay1/1 -> Add12/2, Scope8/7, Product6/2, Out1/1
  Constant1/1 -> Product2/3
  [ILc] -> Add9/1, Scope8/1
  Product2/1 -> Add12/1, Scope8/4

== system shuntconverterlms1/shunt controller/Shunt controller1/Subsystem7 ==
  Add12 : Sum
  Add9 : Sum  Inputs=+-
  Constant1 : Constant  Value=0.001
  Product2 : Product  Inputs=3
  Product6 : Product
  Scope8 : Scope  NumInputPorts=7
  Unit Delay1 : UnitDelay  SampleTime=10e-6  HasFrameUpgradeWarning=on
  Out1 : Outport
  wires:
  Product2/1 -> Scope8/4, Add12/1
  [ILa] -> Add9/1
  Constant1/1 -> Product2/3
  Unit Delay1/1 -> Out1/1, Product6/2, Scope8/7, Add12/2
  Add12/1 -> Unit Delay1/1
  [jpa] -> Product6/1
  Add9/1 -> Product2/2
  Product6/1 -> Add9/2
  [jpa] -> Product2/1
